simulink model "tempTest_PC"  (R2021b)
settings: Solver=FixedStepDiscrete  StartTime=0.0  StopTime=200  FixedStep=0.005  RelTol=1e-3
settings Model: Creator=MSI-NB  LastModifiedBy=MSI-NB

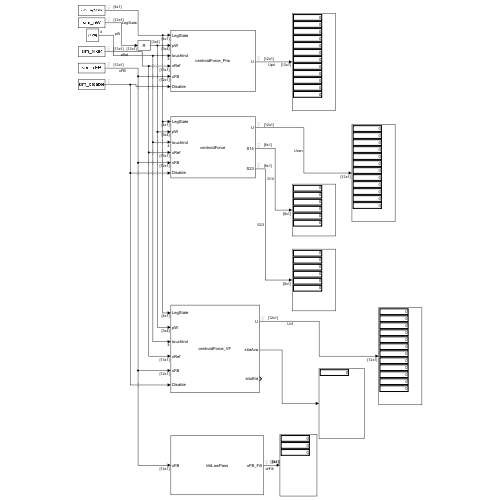
[thumbnail: Simulink's stored preview of the top-level diagram]
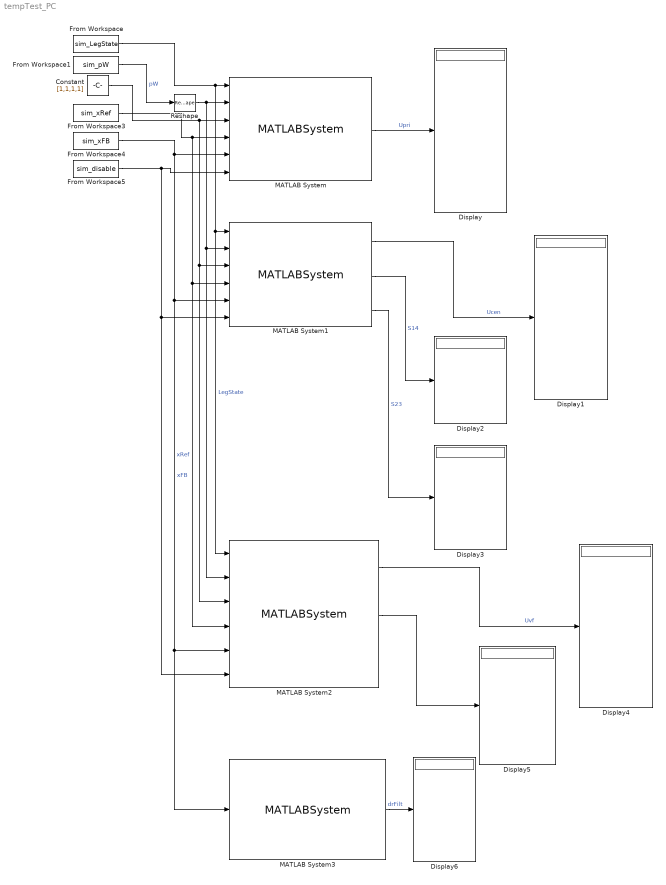
== system tempTest_PC ==
  Constant : Constant  Value=[1,1,1,1]
  Display{,1..6} (7 alike) : Display
  From Workspace : FromWorkspace  VariableName=sim_LegState  SampleTime=0.005
  From Workspace1 : FromWorkspace  VariableName=sim_pW  SampleTime=0.005
  From Workspace3 : FromWorkspace  VariableName=sim_xRef  SampleTime=0.005
  From Workspace4 : FromWorkspace  VariableName=sim_xFB  SampleTime=0.005
  From Workspace5 : FromWorkspace  VariableName=sim_disable  SampleTime=0.005
  MATLAB System : MATLABSystem  System=centroidForce_Prio  krz=1  kpit=1  krol=1  kyaw=1  kwx=0.001  kwy=0.001  Inorm=diag( [0.0046125 0.0230942 0.0253262] )  Ts=0.005  SimulateUsing=Code generation
      mask Type: centroidForce_Prio
      mask Display:
      | disp('centroidForce_Prio');
      | port_label('input',1,'LegState');
      | port_label('input',2,'pW');
      | port_label('input',3,'touchInd');
      | port_label('input',4,'xRef');
      | port_label('input',5,'xFB');
      | port_label('input',6,'Disable');
      | port_label('output',1,'U');
  MATLAB System1 : MATLABSystem  System=centroidForce  kp="[0,  0,  0,  60,  60,  0]"  kd=zeros( 1, 6 )  ki="[0,  0,  0,  0.02,  0.001,  0]"  Inorm=diag( [0.0046125 0.0230942 0.0253262] )  Ts=0.005  SimulateUsing=Interpreted execution
      mask Type: centroidForce
      mask Display:
      | disp('centroidForce');
      | port_label('input',1,'LegState');
      | port_label('input',2,'pW');
      | port_label('input',3,'touchInd');
      | port_label('input',4,'xRef');
      | port_label('input',5,'xFB');
      | port_label('input',6,'Disable');
      | port_label('output',1,'U');
      | port_label('output',2,'S14');
      | port_label('output',3,'S23');
  MATLAB System2 : MATLABSystem  System=centroidForce_VF  kp=[0,0,0,30,40,0]  kd=[0,0,0,0,0,0]  ki=[0,0,0,0,0,0]  SimulateUsing=Code generation
      mask Type: centroidForce_VF
      mask Display:
      | disp('centroidForce_VF');
      | port_label('input',1,'LegState');
      | port_label('input',2,'pW');
      | port_label('input',3,'touchInd');
      | port_label('input',4,'xRef');
      | port_label('input',5,'xFB');
      | port_label('input',6,'Disable');
      | port_label('output',1,'U');
      | port_label('output',2,'sitaAva');
      | port_label('output',3,'sitaStd');
  MATLAB System3 : MATLABSystem  System=VelLowPass  filtN=90  SimulateUsing=Code generation
      mask Type: VelLowPass
      mask Display:
      | disp('VelLowPass');
      | port_label('input',1,'xFB');
      | port_label('output',1,'xFB_Filt');
  Reshape : Reshape  OutputDimensionality=Customize  OutputDimensions=[3,4]
  wires:
  MATLAB System/1 -> Display/1  "Upri"
  From Workspace/1 -> MATLAB System2/1, MATLAB System1/1, MATLAB System/1  "LegState"
  From Workspace1/1 -> Reshape/1  "pW"
  Constant/1 -> MATLAB System2/3, MATLAB System1/3, MATLAB System/3
  From Workspace3/1 -> MATLAB System2/4, MATLAB System1/4, MATLAB System/4  "xRef"
  From Workspace4/1 -> MATLAB System3/1, MATLAB System2/5, MATLAB System1/5, MATLAB System/5  "xFB"
  From Workspace5/1 -> MATLAB System2/6, MATLAB System1/6, MATLAB System/6
  Reshape/1 -> MATLAB System2/2, MATLAB System1/2, MATLAB System/2
  MATLAB System1/1 -> Display1/1  "Ucen"
  MATLAB System1/2 -> Display2/1  "S14"
  MATLAB System1/3 -> Display3/1  "S23"
  MATLAB System2/1 -> Display4/1  "Uvf"
  MATLAB System2/2 -> Display5/1
  MATLAB System3/1 -> Display6/1  "drFilt"
